simulink model "ArUcoSampleModel"  (R2020a)
settings: Solver=FixedStepAuto  StartTime=0.0  StopTime=Inf  RelTol=1e-3  EnableMultiTasking=on
libraries: embdlinuxlib x1
settings Model: Creator=eisuk  LastModifiedBy=eisuk
settings SolverCC: PositivePriorityOrder=on
settings DataIOCC: ReturnWorkspaceOutputs=off
settings OptimizationCC: EnhancedBackFolding=on  PassReuseOutputArgsAs=Individual arguments  ZeroExternalMemoryAtStartup=off  ZeroInternalMemoryAtStartup=off  MaxStackSize=64  OptimizeBlockOrder=speed  DifferentSizesBufferReuse=on  OptimizationCustomize=off  EfficientTunableParamExpr=on
settings DebuggingCC: ParameterTunabilityLossMsg=error
settings HardwareCC: ProdBitPerPointer=32  ProdBitPerSizeT=32  ProdBitPerPtrDiffT=32  ProdLargestAtomicInteger=Long  ProdLargestAtomicFloat=Double  ProdWordSize=32  ProdLongLongMode=on  ProdHWDeviceType=ARM Compatible->ARM Cortex
settings RTWCC: SystemTargetFile=ert.tlc  HardwareBoard=Raspberry Pi  TemplateMakefile=ert_default_tmf  Toolchain=GNU GCC Raspberry Pi  BuildConfiguration=Faster Runs  TargetLang=C++
settings CodeAppCC: ForceParamTrailComments=on  IgnoreCustomStorageClasses=off  OperatorAnnotations=on  SimulinkDataObjDesc=on  SFDataObjDesc=on  InsertBlockDesc=on
settings ERTTargetCC: TargetLangStandard=C++03 (ISO)  SupportVariableSizeSignals=on

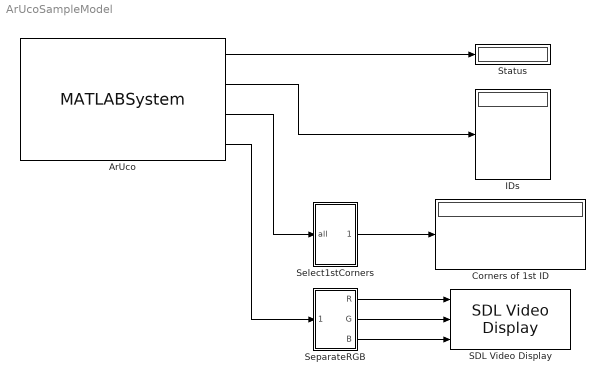
== system ArUcoSampleModel ==
  ArUco : MATLABSystem  System=aruco_raspi_wrapper  markLength=0.1  dictionary=DICT_ARUCO_ORIGINAL  samplingTime=0.2  arraySize=5  isOutCorners=on  isOutVectors=off  isOutImage=on  camSource=0  calibFile=/home/pi/calibration.yml  capWidth=640  capHeight=480
      mask Type: aruco_raspi_wrapper
      mask Display:
      | disp(['ArUco\nMarkerDetection' char(10) '' char(10) 'Marker length: 0.1 m' char(10) 'Dictionary: \nDICT_ARUCO_ORIGINAL' char(10) 'Dimension: 640 x 480']);
      | port_label('output',1,'status');
      | port_label('output',2,'ids');
      | port_label('output',3,'corners');
      | port_label('output',4,'image');
  Corners of 1st ID : Display
  IDs : Display
  SDL Video Display : embdlinuxlib/SDL Video Display  pixelFormat=RGB  pixelOrder=Planar  rowMajor=on  blockPlatform=Raspberry Pi
      settings: SourceProductBaseCode=SC_BEAGLEBONE_BLUE,RASPPI
  Select1stCorners : Subsystem
  SeparateRGB : Subsystem
  Status : Display
  wires:
  Select1stCorners/1(first) -> Corners of 1st ID/1
  ArUco/3 -> Select1stCorners/1(all)
  SeparateRGB/3(B) -> SDL Video Display/3
  SeparateRGB/2(G) -> SDL Video Display/2
  SeparateRGB/1(R) -> SDL Video Display/1
  ArUco/4 -> SeparateRGB/1(RGB)
  ArUco/1 -> Status/1
  ArUco/2 -> IDs/1

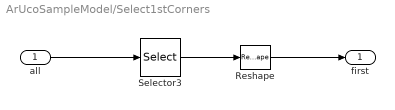
== system ArUcoSampleModel/Select1stCorners ==
  all : Inport
  Reshape : Reshape  OutputDimensionality=Customize  OutputDimensions=[4,2]
  Selector3 : Selector  NumberOfDimensions=3  InputPortWidth=3  IndexOptions=Index vector (dialog),Select all,Select all  Indices=1,[1:5],1  OutputSizes=1,1,1
  first : Outport
  wires:
  Reshape/1 -> first/1
  Selector3/1 -> Reshape/1
  all/1 -> Selector3/1

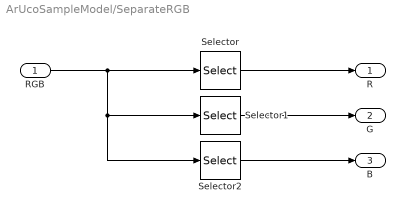
== system ArUcoSampleModel/SeparateRGB ==
  RGB : Inport
  Selector : Selector  NumberOfDimensions=3  InputPortWidth=3  IndexOptions=Select all,Select all,Index vector (dialog)  Indices=[1:5],[1:5],1  OutputSizes=1,1,1
  Selector1 : Selector  NumberOfDimensions=3  InputPortWidth=3  IndexOptions=Select all,Select all,Index vector (dialog)  Indices=[1 3],1,2  OutputSizes=1,1,1
  Selector2 : Selector  NumberOfDimensions=3  InputPortWidth=3  IndexOptions=Select all,Select all,Index vector (dialog)  Indices=[1 3],1,3  OutputSizes=1,1,1
  R : Outport
  G : Outport  Port=2
  B : Outport  Port=3
  wires:
  Selector1/1 -> G/1
  Selector/1 -> R/1
  Selector2/1 -> B/1
  RGB/1 -> Selector/1, Selector1/1, Selector2/1
